simulink model "control_system"  (R2020b)
settings: Solver=FixedStepAuto  StartTime=0.0  StopTime=t_sim  FixedStep=Ts  RelTol=1e-2
values from neighbouring files (symbols this model uses):
  Hp = 10    [main_script.m]
  InitPosX = -2.4980e+03    (= -2498)    [main_script.m]
  InitPosY = -650.5503    [main_script.m]
  InitVelX = V0*cosd(InitYaw)    [main_script.m]
  InitVelY = V0*sind(InitYaw)    [main_script.m]
  InitYaw = 21    [main_script.m]
  lr = 1.592    [main_script.m]
  m = 1625    [main_script.m]
  Ts = 0.1    [main_script.m]
  V0 = 25    [main_script.m]
libraries: neural x856, simulink x1, autolibshared x1, drivingscenarioandsensors x1
(part 23 of 40)

== system control_system/50 30 2+3+4+5+6+7+8+9+16+17 ok rett 100 - 108 /Layer 3/Delays 1 ==
  "p{3}" : Inport  PortDimensions=30  SampleTime=0.1
      mask Display: e = 0.06;c1 = [120 230 180]/255;c2 = ([120 230 180]+0)/(256+128);c3 = ([120 230 180]+128)/(256+128);patch([0 1 1 0],[0 0 1 1],c1);patch([0 1 1 1-e 1-e 0+e],[0 0 1 1-e 0+e 0+e],c2);patch([0 0 1 1-e 0+e 0+e],[0 1 1 1-e 1-e 0+e],c3);plot([0 1 1 0 0],[0 0 1 1 0]);
  mux : Mux  Inputs=1
      mask Display: e = 0.06;c1 = [120 150 230]/255;c2 = ([120 150 230]+0)/383;c3 = ([120 150 230]+128)/383;patch([0 1 1 0],[0 0 1 1],c1);patch([0 1 1 1-e 1-e 0+e],[0 0 1 1-e 0+e 0+e],c2);patch([0 0 1 1-e 0+e 0+e],[0 1 1 1-e 1-e 0+e],c3);plot([0 1 1 0 0],[0 0 1 1 0]);disp('Mux')
  "pd{3,2}" : Outport
      mask Display: e = 0.06;c1 = [120 230 180]/255;c2 = ([120 230 180]+0)/(256+128);c3 = ([120 230 180]+128)/(256+128);patch([0 1 1 0],[0 0 1 1],c1);patch([0 1 1 1-e 1-e 0+e],[0 0 1 1-e 0+e 0+e],c2);patch([0 0 1 1-e 0+e 0+e],[0 1 1 1-e 1-e 0+e],c3);plot([0 1 1 0 0],[0 0 1 1 0]);
  wires:
  "p{3}"/1 -> mux/1
  mux/1 -> "pd{3,2}"/1

== system control_system/50 30 2+3+4+5+6+7+8+9+16+17 ok rett 100 - 108 /Layer 3/LW{3,2} ==
  "ad{3,2}" : Inport  PortDimensions=30  SampleTime=0.1
      mask Display: e = 0.06;c1 = [120 230 180]/255;c2 = ([120 230 180]+0)/(256+128);c3 = ([120 230 180]+128)/(256+128);patch([0 1 1 0],[0 0 1 1],c1);patch([0 1 1 1-e 1-e 0+e],[0 0 1 1-e 0+e 0+e],c2);patch([0 0 1 1-e 0+e 0+e],[0 1 1 1-e 1-e 0+e],c3);plot([0 1 1 0 0],[0 0 1 1 0]);
  "IW{3,2}(1,:)'" : Constant  Value=[0.5875934491844534424132007188745774328708648681640625;-1.5303503248291792093738195035257376730442047119140625;-0.06067190872641288479361065810735453851521015167236328125;-1.71048463570641917641523832571692764759063720703125;3.042670458649316511667848317301832139492034912109375;-1.6475294245005418503069449798204004764556884765625;2.66537911112479708464206851203925907611846923828125;2.134528428679815181823187231202609837055206298828125;-0.44149350097525330571812673952081240713596343994140625;-1.0305811868557521737699289587908424437046051025390625;0.78547825539922355719824054176569916307926177978515625;1.7344610647341498488316346993087790906429290771484375;3.242670436715069381961029648664407432079315185546875;-1.85472957250165659814911123248748481273651123046875;0.499277820201845023984077442946727387607097625732421875;-0.5169053091276847311519304639659821987152099609375;-1.3061971584850551320045042302808724343776702880859375;2.03099658823449846778430583071894943714141845703125;-2.329665421258628299483461887575685977935791015625;-0.98742547665986635241353042147238738834857940673828125;2.015772987252038905836570847895927727222442626953125;1.7608701120573180265438395508681423962116241455078125;-2.482123069568679785135145721142180263996124267578125;0.926032886701367630166714661754667758941650390625;-2.17633179100425255825257409014739096164703369140625;-1.71056121012020145855103692156262695789337158203125;0.78764512038736411714268115247250534594058990478515625;1.73071785927034937913049361668527126312255859375;-1.7391896088638165718265327086555771529674530029296875;0.67915043807232666761564132684725336730480194091796875]
      mask Display: e = 0.06;c1 = [120 150 230]/255;c2 = ([120 150 230]+0)/383;c3 = ([120 150 230]+128)/383;patch([0 1 1 0],[0 0 1 1],c1);patch([0 1 1 1-e 1-e 0+e],[0 0 1 1-e 0+e 0+e],c2);patch([0 0 1 1-e 0+e 0+e],[0 1 1 1-e 1-e 0+e],c3);plot([0 1 1 0 0],[0 0 1 1 0]);disp('weights');
  Mux : Mux  Inputs=1
      mask Display: e = 0.06;c1 = [120 150 230]/255;c2 = ([120 150 230]+0)/383;c3 = ([120 150 230]+128)/383;patch([0 1 1 0],[0 0 1 1],c1);patch([0 1 1 1-e 1-e 0+e],[0 0 1 1-e 0+e 0+e],c2);patch([0 0 1 1-e 0+e 0+e],[0 1 1 1-e 1-e 0+e],c3);plot([0 1 1 0 0],[0 0 1 1 0]);disp('Mux');
  dotprod1 : neural/Weight Functions/dotprod
  "lz{3,2}" : Outport
      mask Display: e = 0.06;c1 = [120 230 180]/255;c2 = ([120 230 180]+0)/(256+128);c3 = ([120 230 180]+128)/(256+128);patch([0 1 1 0],[0 0 1 1],c1);patch([0 1 1 1-e 1-e 0+e],[0 0 1 1-e 0+e 0+e],c2);patch([0 0 1 1-e 0+e 0+e],[0 1 1 1-e 1-e 0+e],c3);plot([0 1 1 0 0],[0 0 1 1 0]);
  wires:
  "IW{3,2}(1,:)'"/1 -> dotprod1/1
  "ad{3,2}"/1 -> dotprod1/2
  dotprod1/1 -> Mux/1
  Mux/1 -> "lz{3,2}"/1

== system control_system/Function Fitting Neural Network/Layer 1/Delays 1 ==
  "p{1}" : Inport  PortDimensions=9  SampleTime=0.1
      mask Display: e = 0.06;c1 = [120 230 180]/255;c2 = ([120 230 180]+0)/(256+128);c3 = ([120 230 180]+128)/(256+128);patch([0 1 1 0],[0 0 1 1],c1);patch([0 1 1 1-e 1-e 0+e],[0 0 1 1-e 0+e 0+e],c2);patch([0 0 1 1-e 0+e 0+e],[0 1 1 1-e 1-e 0+e],c3);plot([0 1 1 0 0],[0 0 1 1 0]);
  mux : Mux  Inputs=1
      mask Display: e = 0.06;c1 = [120 150 230]/255;c2 = ([120 150 230]+0)/383;c3 = ([120 150 230]+128)/383;patch([0 1 1 0],[0 0 1 1],c1);patch([0 1 1 1-e 1-e 0+e],[0 0 1 1-e 0+e 0+e],c2);patch([0 0 1 1-e 0+e 0+e],[0 1 1 1-e 1-e 0+e],c3);plot([0 1 1 0 0],[0 0 1 1 0]);disp('Mux')
  "pd{1,1}" : Outport
      mask Display: e = 0.06;c1 = [120 230 180]/255;c2 = ([120 230 180]+0)/(256+128);c3 = ([120 230 180]+128)/(256+128);patch([0 1 1 0],[0 0 1 1],c1);patch([0 1 1 1-e 1-e 0+e],[0 0 1 1-e 0+e 0+e],c2);patch([0 0 1 1-e 0+e 0+e],[0 1 1 1-e 1-e 0+e],c3);plot([0 1 1 0 0],[0 0 1 1 0]);
  wires:
  "p{1}"/1 -> mux/1
  mux/1 -> "pd{1,1}"/1
